simulink model "FeedbackDiUscitaSimulink"  (R2020b)
settings: Solver=VariableStepAuto  StartTime=0.0  StopTime=10.0  RelTol=1e-3
values from neighbouring files (symbols this model uses):
  A = [-0.0558 -0.9968 0.0802 0.0415; 0.5980 -0.1150 -0.0318 0; -3.0500 0.3880 -0.4650 0; 0 0.0805 1 0]    [AircraftPaper.m]    (also in EsercizioAereo.m = [0 1 0; 0 -.875 -20; 0 0 -50]; FeedbackDiStato.m = [0 1 0; 0 -.875 -20; 0 0 -50]; FeedbackDiUscita.m = [0 1 0; 0 -.875 -20; 0 0 -50]; SetPoint.m = [0 1 0; 0 -.875 -20; 0 0 -50])
  B = [0.0729 0; -4.7500 0.00775; 0.153 0.143; 0 0]    [AircraftPaper.m]    (also in EsercizioAereo.m = [0 0 50]'; FeedbackDiStato.m = [0 0 50]'; FeedbackDiUscita.m = [0 0 50]'; SetPoint.m = [0 0 50]')
  C = [1 0 0 0; 0 0 0 1]    [AircraftPaper.m]    (also in EsercizioAereo.m = [1 0 0; 0 1 0; 0 0 1]; FeedbackDiStato.m = [1 0 0]; FeedbackDiUscita.m = [1 0 0]; SetPoint.m = [1 0 0])
  D = 0    [AircraftPaper.m]    (also in EsercizioAereo.m = [0 0 0]'; FeedbackDiStato.m; FeedbackDiUscita.m; SetPoint.m)
  Kc = lqr(A,B,Q,R)    [AircraftPaper.m]    (also in EsercizioAereo.m; FeedbackDiStato.m; FeedbackDiUscita.m = lqr(A,B,Qc,Rc); SetPoint.m = lqr(A,B,Qc,Rc))
  x0 = [1 1 1]'    [EsercizioAereo.m]    (also in FeedbackDiStato.m; FeedbackDiUscita.m = [1 1 1]; SetPoint.m = [1 1 1]; SetPointProf.m = [0 0 ]')
libraries: cstblocks x1
settings Model: Creator=leobartowski  LastModifiedBy=leobartowski

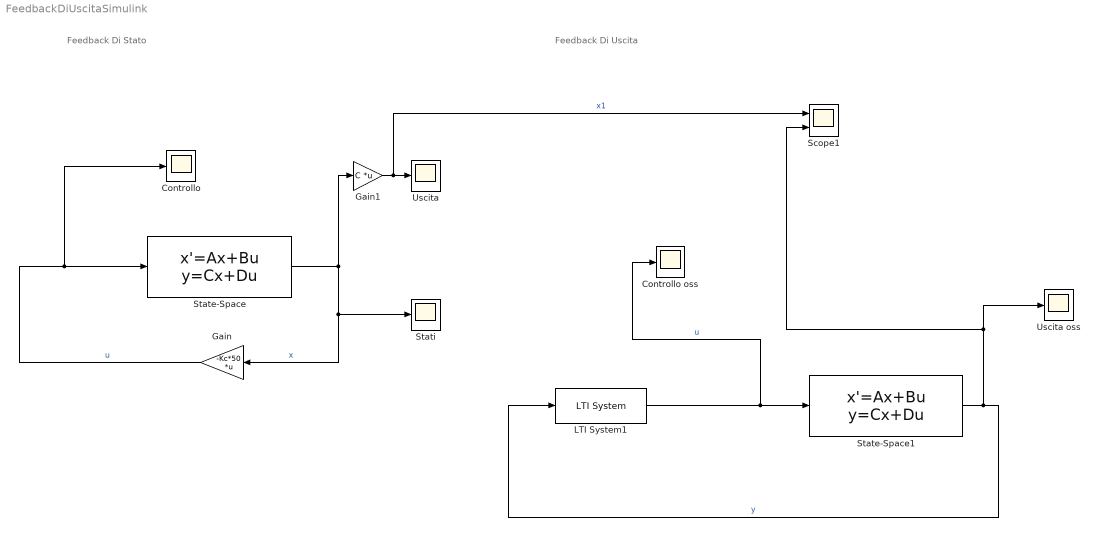
== system FeedbackDiUscitaSimulink ==
  note: Feedback Di Stato
  note: Feedback Di Uscita
  Controllo : Scope
  Controllo oss : Scope
  Gain : Gain  Gain=-Kc*50  Multiplication=Matrix(K*u)
  Gain1 : Gain  Gain=C  Multiplication=Matrix(K*u)
  LTI System1 : cstblocks/LTI System  sys=K  IC=[]
  Scope1 : Scope  NumInputPorts=2
  State-Space : StateSpace  A=A  B=B  C=eye(3)  D=zeros(3,1)  InitialCondition=x0
  State-Space1 : StateSpace  A=A  B=B  C=C  D=D  InitialCondition=x0
  Stati : Scope
  Uscita : Scope
  Uscita oss : Scope
  wires:
  State-Space/1 -> Gain1/1, Gain/1, Stati/1  "x"
  Gain/1 -> Controllo/1, State-Space/1  "u"
  Gain1/1 -> Scope1/1, Uscita/1  "x1"
  LTI System1/1 -> Controllo oss/1, State-Space1/1  "u"
  State-Space1/1 -> Scope1/2, Uscita oss/1, LTI System1/1  "y"
